simulink model "Lab_1_simulink"  (R2022b)
settings: Solver=VariableStepAuto  StartTime=0.0  StopTime=10.0  RelTol=1e-3
undefined symbols (not defined in the file or in its folder): a1, c1, h10
settings Model: Creator=Gabriel  LastModifiedBy=barte
settings DataIOCC: ReturnWorkspaceOutputs=off

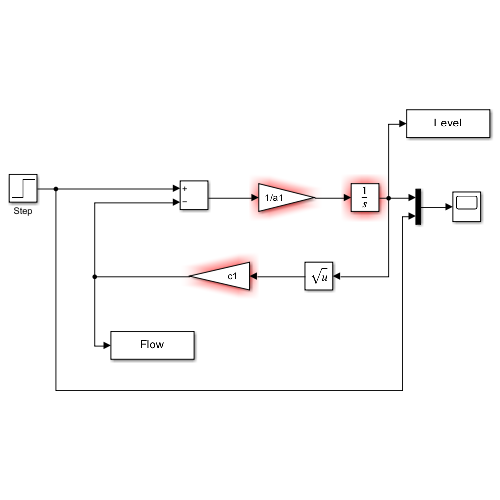
[thumbnail: Simulink's stored preview of the top-level diagram]
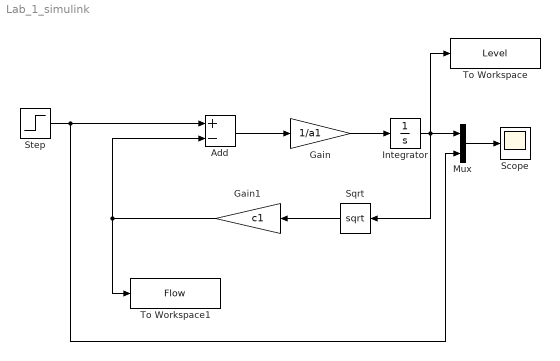
== system Lab_1_simulink ==
  Add : Sum  Inputs=+-
  Gain : Gain  Gain=1/a1
  Gain1 : Gain  Gain=c1
  Integrator : Integrator  InitialCondition=h10
  Mux : Mux  Inputs=2
  Scope : Scope
  Sqrt : Sqrt
  Step : Step  Time=0  SampleTime=0
  To Workspace : ToWorkspace  VariableName=Level  SaveFormat=Timeseries  SampleTime=-1
  To Workspace1 : ToWorkspace  VariableName=Flow  SaveFormat=Timeseries  SampleTime=-1
  wires:
  Step/1 -> Mux/2, Add/1
  Add/1 -> Gain/1
  Gain/1 -> Integrator/1
  Integrator/1 -> Sqrt/1, Mux/1, To Workspace/1
  Mux/1 -> Scope/1
  Sqrt/1 -> Gain1/1
  Gain1/1 -> To Workspace1/1, Add/2
